simulink model "Performance"  (R2019b)
settings: Solver=VariableStepAuto  StartTime=0.0  StopTime=0.8  RelTol=1e-3
undefined symbols (not defined in the file): DiscIntNeverNeededParam
libraries: dsparch4 x1, commsynccomp2 x1, dspsrcs4 x1
settings Model: Creator=Dell  LastModifiedBy=Dell

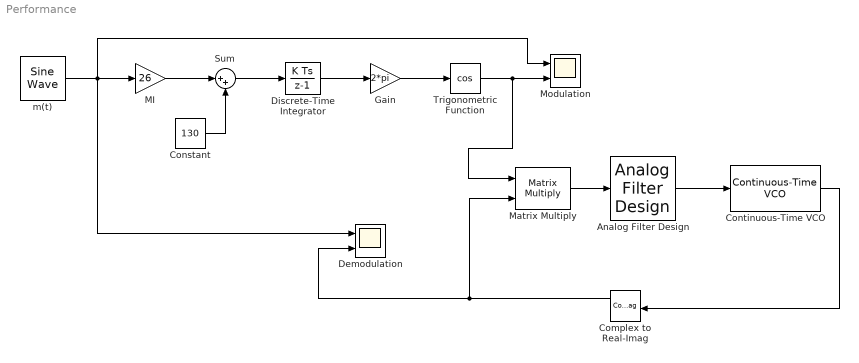
== system Performance ==
  "Analog Filter Design " : dsparch4/Analog Filter Design  method=Butterworth  filttype=Lowpass  N=8  Wlo=30  Whi=80  Rp=2  Rs=40
  "Complex to Real-Imag " : ComplexToRealImag
  Constant : Constant  Value=130
  "Continuous-Time VCO " : commsynccomp2/Continuous-Time VCO  Ac=1  Fc=10  Kc=1  Ph=0
      settings: SourceProductName=Communications Toolbox  SourceProductBaseCode=CM
  "Demodulation " : Scope  NumInputPorts=2
  "Discrete-Time Integrator " : DiscreteIntegrator  InitialCondition=1/10000  SampleTime=-1  ICPrevOutput=DiscIntNeverNeededParam  ICPrevScaledInput=DiscIntNeverNeededParam
  "Gain " : Gain  Gain=2*pi
  "MI " : Gain  Gain=26
  "Matrix Multiply " : Product  Multiplication=Matrix(*)
  "Modulation " : Scope  NumInputPorts=2
  Sum : Sum  Inputs=|++
  "Trigonometric Function " : Trigonometry  Operator=cos
  "m(t) " : dspsrcs4/Sine Wave  Amplitude=13  Frequency=3  Phase=60  SampleMode=Discrete  OutComplex=Real  CompMethod=Trigonometric fcn  TableSize=Speed  SampleTime=1/98000  SamplesPerFrame=1  ResetState=Restart at time zero  OutputFrames=off  dataType=double  wordLen=16  udDataType=sfix(16)  fracBitsMode=Best precision  numFracBits=15  OutDataTypeStr=double  LastOutDataTypeStr=double
  wires:
  "MI "/1 -> Sum/1
  Sum/1 -> "Discrete-Time Integrator "/1
  "Discrete-Time Integrator "/1 -> "Gain "/1
  "Gain "/1 -> "Trigonometric Function "/1
  "Trigonometric Function "/1 -> "Matrix Multiply "/1, "Modulation "/2
  Constant/1 -> Sum/2
  "Matrix Multiply "/1 -> "Analog Filter Design "/1
  "Analog Filter Design "/1 -> "Continuous-Time VCO "/1
  "Continuous-Time VCO "/1 -> "Complex to Real-Imag "/1
  "Complex to Real-Imag "/1 -> "Demodulation "/2, "Matrix Multiply "/2
  "m(t) "/1 -> "MI "/1, "Modulation "/1, "Demodulation "/1
